simulink model "DC-Motor_simulation1"  (R2020a)
settings: Solver=VariableStepAuto  StartTime=0.0  StopTime=10.0  RelTol=1e-3
libraries: arduinolib x3
settings Model: Creator=junio  LastModifiedBy=junio

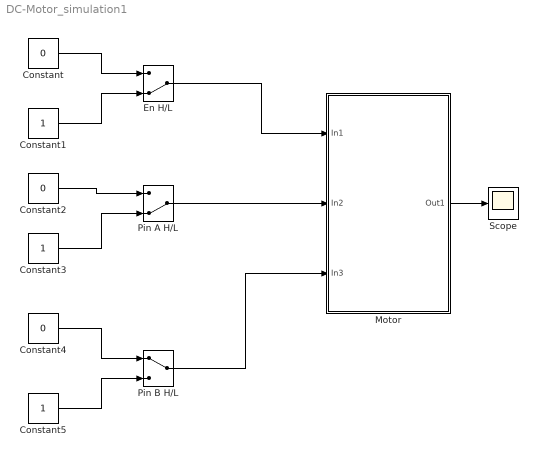
== system DC-Motor_simulation1 ==
  Constant : Constant  Value=0
  Constant1 : Constant
  Constant2 : Constant  Value=0
  Constant3 : Constant
  Constant4 : Constant  Value=0
  Constant5 : Constant
  En H/L : ManualSwitch  CurrentSetting=0
  Motor : Subsystem
  Pin A H/L : ManualSwitch  CurrentSetting=0
  Pin B H/L : ManualSwitch
  Scope : Scope
  wires:
  Constant/1 -> En H/L/1
  Constant1/1 -> En H/L/2
  Constant2/1 -> Pin A H/L/1
  Constant3/1 -> Pin A H/L/2
  Constant4/1 -> Pin B H/L/1
  Constant5/1 -> Pin B H/L/2
  En H/L/1 -> Motor/1(In1)
  Pin A H/L/1 -> Motor/2(In2)
  Pin B H/L/1 -> Motor/3(In3)
  Motor/1(Out1) -> Scope/1

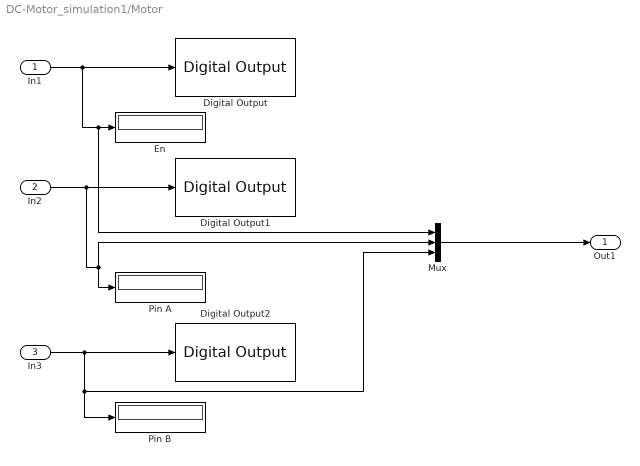
== system DC-Motor_simulation1/Motor ==
  In1 : Inport
  In2 : Inport  Port=2
  In3 : Inport  Port=3
  Digital Output : arduinolib/Digital Output  pinNumber=9  Direction=output  blockPlatform=arduino
  Digital Output1 : arduinolib/Digital Output  pinNumber=10  Direction=output  blockPlatform=arduino
  Digital Output2 : arduinolib/Digital Output  pinNumber=11  Direction=output  blockPlatform=arduino
  En : Display
  Mux : Mux  Inputs=3
  Pin A : Display
  Pin B : Display
  Out1 : Outport
  wires:
  In2/1 -> Mux/2, Pin A/1, Digital Output1/1
  In3/1 -> Mux/3, Pin B/1, Digital Output2/1
  In1/1 -> Mux/1, En/1, Digital Output/1
  Mux/1 -> Out1/1
